simulink model "second"  (R2020b)
settings: Solver=VariableStepAuto  StartTime=0.0  StopTime=10.0  RelTol=1e-3
undefined symbols (not defined in the file): k1, m1, m2
settings Model: Creator=priyaD  LastModifiedBy=priyaD

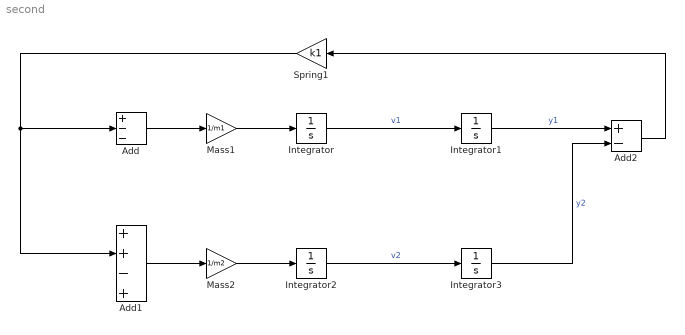
== system second ==
  Add : Sum  Inputs=+--
  Add1 : Sum  Inputs=++-+
  Add2 : Sum  Inputs=+-
  Integrator{,1..3} (4 alike) : Integrator
  Mass1 : Gain  Gain=1/m1
  Mass2 : Gain  Gain=1/m2
  Spring1 : Gain  Gain=k1
  wires:
  Integrator/1 -> Integrator1/1  "v1"
  Integrator2/1 -> Integrator3/1  "v2"
  Integrator1/1 -> Add2/1  "y1"
  Integrator3/1 -> Add2/2  "y2"
  Mass1/1 -> Integrator/1
  Mass2/1 -> Integrator2/1
  Add/1 -> Mass1/1
  Add1/1 -> Mass2/1
  Add2/1 -> Spring1/1
  Spring1/1 -> Add/2, Add1/2
